simulink model "sensor_test"  (R2024a)
settings: Solver=FixedStepAuto  StartTime=0.0  StopTime=inf  FixedStep=0.01  RelTol=1e-3  EnableMultiTasking=on
InitFcn:
  | measRate = 0.01;
  | alpha = 0.98;
libraries: hdlsllib x6, simulink x6
settings Model: STM32="{\"I2CControllerRead\":[{\"ID\":\"sensor_test:45\"},{\"ID\":\"sensor_test:29\"},{\"ID\":\"sensor_test:30\"},{\"ID\":\"sensor_test:89\"},{\"ID\":\"sensor_test:122\"},{\"ID\":\"sensor_test:123\"},{\"ID\":\"sensor_test:124\"},{\"ID\":\"sensor_test:199\"},{\"ID\":\"sensor_test:214:7\"},{\"ID\":\"sensor_test:214:18\"},{\"ID\":\"sensor_test:214:19\"},{\"ID\":\"sensor_test:214:20\"},{\"ID\":\"sensor_test:206:7\"},{\"ID\":\"sensor_test:206:15\"},{\"ID\":\"sensor_test:206:16\"},{\"ID\":\"sensor_test:206:17\"}],\"I2CControllerWrite\":[{\"ID\":\"sensor_test:31\"},{\"ID\":\"sensor_test:32\"},{\"ID\":\"sensor_test:90\"},{\"ID\":\"sensor_test:125\"},{\"ID\":\"sensor_test:126\"},{\"ID\":\"sensor_test:127\"},{\"ID\":\"sensor_test:214:21\"},{\"ID\":\"sensor_test:214:22\"},{\"ID\":\"sensor_test:214:23\"},{\"ID\":\"sensor_test:206:18\"},{\"ID\":\"sensor_test:206:19\"},{\"ID\":\"sensor_test:206:20\"}]}"  Creator=Peter  LastModifiedBy=Peter
settings OptimizationCC: EnhancedBackFolding=on  PassReuseOutputArgsAs=Individual arguments  ZeroExternalMemoryAtStartup=off  ZeroInternalMemoryAtStartup=off  MaxStackSize=64  OptimizeBlockOrder=speed  DifferentSizesBufferReuse=on  OptimizationCustomize=off  EfficientTunableParamExpr=on
settings DebuggingCC: ParameterTunabilityLossMsg=error
settings HardwareCC: ProdBitPerPointer=32  ProdBitPerSizeT=32  ProdBitPerPtrDiffT=32  ProdLargestAtomicInteger=Long  ProdLargestAtomicFloat=Double  ProdWordSize=32  ProdLongLongMode=on  ProdHWDeviceType=ARM Compatible->ARM Cortex-M
settings SFSimCC: MATLABDynamicMemAlloc=off
settings RTWCC: Description=Embedded Coder  SystemTargetFile=ert.tlc  HardwareBoard=STM32F7xx Based (Single precision FPU)  TemplateMakefile=ert_default_tmf  Toolchain=GNU Tools for ARM Embedded Processors
settings CodeAppCC: ForceParamTrailComments=on  IgnoreCustomStorageClasses=off  OperatorAnnotations=on  SimulinkDataObjDesc=on  SFDataObjDesc=on  InsertBlockDesc=on
settings ERTTargetCC: TargetLangStandard=C99 (ISO)  CodeReplacementLibrary=ARM Cortex-M  ExtModeTransport=3  ExtModeStaticAlloc=on  ExtModeStaticAllocSize=2048  ExtModeMexFile=ext_xcp  ExtModeIntrfLevel=Level2 - Open

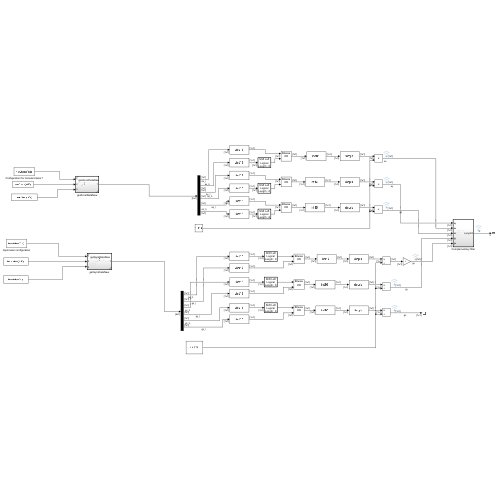
[thumbnail: Simulink's stored preview of the top-level diagram]
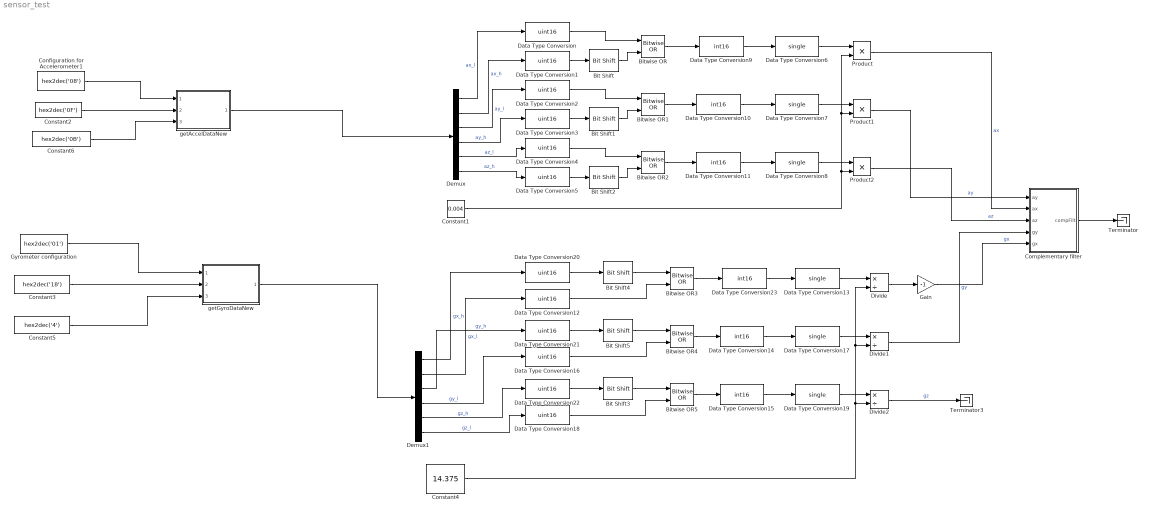
== system sensor_test ==
  Bit Shift{,1..5} (6 alike) : hdlsllib/Logic and Bit Operations/Bit Shift  mode=Shift Left Logical  N=8
  Bitwise OR{,1..5} (6 alike) : simulink/Logic and Bit Operations/Bitwise Operator  logicop=OR  UseBitMask=off  NumInputPorts=2  BitMask=bin2dec('11011001')  BitMaskRealWorld=Stored Integer
      settings: LibrarySourceBlock=|
      | simulink/Quick Insert/Logic and Bit
      | Operations/Bitwise OR
  Complementary filter : Subsystem  TreatAsAtomicUnit=on  SystemSampleTime=measRate
  Configuration for Accelerometer1 : Constant  Value=hex2dec('08')  OutDataTypeStr=uint8
  Constant1 : Constant  Value=0.004  OutDataTypeStr=single
  Constant2 : Constant  Value=hex2dec('0F')  OutDataTypeStr=uint8
  Constant3 : Constant  Value=hex2dec('18')
  Constant4 : Constant  Value=14.375  OutDataTypeStr=single
  Constant5 : Constant  Value=hex2dec('4')
  Constant6 : Constant  Value=hex2dec('0B')  OutDataTypeStr=uint8
  Data Type Conversion{,1..5,12,16,18,20..22} (12 alike) : DataTypeConversion  OutDataTypeStr=uint16  SaturateOnIntegerOverflow=off  RndMeth=Floor
  Data Type Conversion{9..11,14..15,23} (6 alike) : DataTypeConversion  OutDataTypeStr=int16  SaturateOnIntegerOverflow=off  RndMeth=Floor
  Data Type Conversion{6..8,13,17,19} (6 alike) : DataTypeConversion  OutDataTypeStr=single  SaturateOnIntegerOverflow=off  RndMeth=Floor
  Demux : Demux  Outputs=6
  Demux1 : Demux  Outputs=6
  Divide : Product  Inputs=*/
  Divide1 : Product  Inputs=*/
  Divide2 : Product  Inputs=*/
  Gain : Gain  Gain=-1
  Gyrometer configuration : Constant  Value=hex2dec('01')  OutDataTypeStr=uint8
  Product : Product
  Product1 : Product
  Product2 : Product
  Terminator : Terminator
  Terminator3 : Terminator
  getAccelDataNew : Subsystem  TreatAsAtomicUnit=on  ReferencedSubsystem=getAccelDataNew
  getGyroDataNew : Subsystem  TreatAsAtomicUnit=on  ReferencedSubsystem=getGyroDataNew
  wires:
  Data Type Conversion11/1 -> Data Type Conversion8/1
  Bit Shift2/1 -> Bitwise OR2/2
  Demux/3 -> Data Type Conversion2/1  "ay_l"
  Data Type Conversion5/1 -> Bit Shift2/1
  Data Type Conversion10/1 -> Data Type Conversion7/1
  Bitwise OR2/1 -> Data Type Conversion11/1
  Data Type Conversion9/1 -> Data Type Conversion6/1
  Bitwise OR/1 -> Data Type Conversion9/1
  Data Type Conversion2/1 -> Bitwise OR1/1
  Demux/2 -> Data Type Conversion1/1  "ax_h"
  Data Type Conversion8/1 -> Product2/1
  Data Type Conversion6/1 -> Product/1
  Demux/1 -> Data Type Conversion/1  "ax_l"
  Data Type Conversion7/1 -> Product1/1
  Constant1/1 -> Product2/2, Product/2, Product1/2
  Bitwise OR1/1 -> Data Type Conversion10/1
  Data Type Conversion4/1 -> Bitwise OR2/1
  Demux/5 -> Data Type Conversion4/1  "az_l"
  Product2/1 -> Complementary filter/3(az)  "az"
  Bit Shift1/1 -> Bitwise OR1/2
  Demux/4 -> Data Type Conversion3/1  "ay_h"
  Product1/1 -> Complementary filter/1(ay)  "ay"
  Data Type Conversion3/1 -> Bit Shift1/1
  Product/1 -> Complementary filter/2(ax)  "ax"
  Data Type Conversion1/1 -> Bit Shift/1
  Data Type Conversion/1 -> Bitwise OR/1
  Bit Shift/1 -> Bitwise OR/2
  Demux/6 -> Data Type Conversion5/1  "az_h"
  Bit Shift3/1 -> Bitwise OR5/1
  Divide1/1 -> Complementary filter/4(gy)  "gy"
  Bitwise OR5/1 -> Data Type Conversion15/1
  Data Type Conversion23/1 -> Data Type Conversion13/1
  Data Type Conversion16/1 -> Bitwise OR4/2
  Gain/1 -> Complementary filter/5(gx)  "gx"
  Demux1/5 -> Data Type Conversion22/1  "gz_h"
  Bit Shift4/1 -> Bitwise OR3/1
  Data Type Conversion15/1 -> Data Type Conversion19/1
  Data Type Conversion21/1 -> Bit Shift5/1
  Data Type Conversion22/1 -> Bit Shift3/1
  Demux1/1 -> Data Type Conversion20/1  "gx_h"
  Data Type Conversion13/1 -> Divide/1
  Data Type Conversion17/1 -> Divide1/1
  Data Type Conversion12/1 -> Bitwise OR3/2
  Divide2/1 -> Terminator3/1  "gz"
  Demux1/3 -> Data Type Conversion21/1  "gy_h"
  Constant4/1 -> Divide2/2, Divide1/2, Divide/2
  Data Type Conversion19/1 -> Divide2/1
  Divide/1 -> Gain/1
  Data Type Conversion20/1 -> Bit Shift4/1
  Bit Shift5/1 -> Bitwise OR4/1
  Demux1/6 -> Data Type Conversion18/1  "gz_l"
  Bitwise OR4/1 -> Data Type Conversion14/1
  Data Type Conversion14/1 -> Data Type Conversion17/1
  Data Type Conversion18/1 -> Bitwise OR5/2
  Bitwise OR3/1 -> Data Type Conversion23/1
  Demux1/4 -> Data Type Conversion16/1  "gy_l"
  Demux1/2 -> Data Type Conversion12/1  "gx_l"
  Complementary filter/1(compFilt) -> Terminator/1
  Gyrometer configuration/1 -> getGyroDataNew/1
  Constant3/1 -> getGyroDataNew/2
  Constant5/1 -> getGyroDataNew/3
  getGyroDataNew/1 -> Demux1/1
  getAccelDataNew/1 -> Demux/1
  Configuration for Accelerometer1/1 -> getAccelDataNew/1
  Constant2/1 -> getAccelDataNew/2
  Constant6/1 -> getAccelDataNew/3

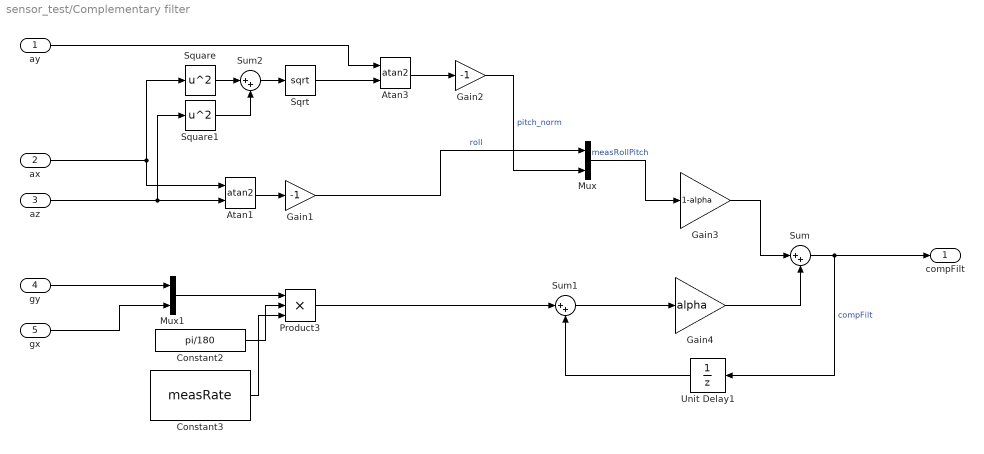
== system sensor_test/Complementary filter ==
  ay : Inport
  ax : Inport  Port=2
  az : Inport  Port=3
  gy : Inport  Port=4
  gx : Inport  Port=5
  Atan1 : Trigonometry  Operator=atan2
  Atan3 : Trigonometry  Operator=atan2
  Constant2 : Constant  Value=pi/180  OutDataTypeStr=single
  Constant3 : Constant  Value=measRate  OutDataTypeStr=single
  Gain1 : Gain  Gain=-1
  Gain2 : Gain  Gain=-1  OutDataTypeStr=single
  Gain3 : Gain  Gain=1-alpha  OutDataTypeStr=single
  Gain4 : Gain  Gain=alpha  OutDataTypeStr=single
  Mux : Mux  Inputs=2
  Mux1 : Mux  Inputs=2
  Product3 : Product  Inputs=3
  Sqrt : Sqrt
  Square : Math  Operator=square
  Square1 : Math  Operator=square
  Sum : Sum  Inputs=|++
  Sum1 : Sum  Inputs=|++
  Sum2 : Sum  Inputs=|++
  Unit Delay1 : UnitDelay  SampleTime=measRate  HasFrameUpgradeWarning=on
  compFilt : Outport
  wires:
  Gain3/1 -> Sum/1
  Sqrt/1 -> Atan3/2
  Atan1/1 -> Gain1/1
  ax/1 -> Atan1/1, Square/1
  Gain4/1 -> Sum/2
  Sum1/1 -> Gain4/1
  Sum/1 -> compFilt/1, Unit Delay1/1  "compFilt"
  Atan3/1 -> Gain2/1
  gy/1 -> Mux1/1
  Mux/1 -> Gain3/1  "measRollPitch"
  Square1/1 -> Sum2/2
  Mux1/1 -> Product3/1
  Square/1 -> Sum2/1
  Constant2/1 -> Product3/2
  Sum2/1 -> Sqrt/1
  Unit Delay1/1 -> Sum1/2
  Gain2/1 -> Mux/2  "pitch_norm"
  az/1 -> Atan1/2, Square1/1
  Constant3/1 -> Product3/3
  Product3/1 -> Sum1/1
  Gain1/1 -> Mux/1  "roll"
  gx/1 -> Mux1/2
  ay/1 -> Atan3/1
